simulink model "segway_PID2"  (R2020a)
settings: Solver=VariableStepAuto  StartTime=0.0  StopTime=60  RelTol=1e-3
undefined symbols (not defined in the file or in its folder): den1, den2, num1, num2
libraries: simulink x5
settings Model: Creator=santi  LastModifiedBy=santi

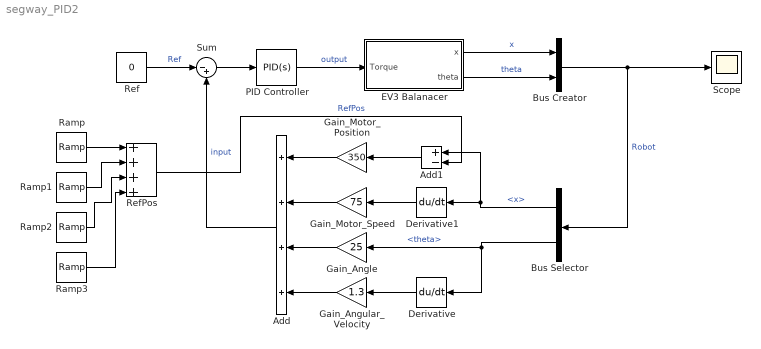
== system segway_PID2 ==
  Add : Sum  Inputs=++++
  Add1 : Sum  Inputs=+-
  Bus Creator : BusCreator  Inputs=2
  Bus Selector : BusSelector  OutputSignals=x,theta
  Derivative : Derivative
  Derivative1 : Derivative
  EV3 Balanacer : Subsystem
  Gain_Angle : Gain  Gain=25
  Gain_Angular_Velocity : Gain  Gain=1.3
  Gain_Motor_Position : Gain  Gain=350
  Gain_Motor_Speed : Gain  Gain=75
  PID Controller : simulink/Continuous/PID Controller  Controller=PID  Form=Parallel  TimeDomain=Continuous-time  UseExternalTs=off  SampleTime=-1  IntegratorMethod=Forward Euler  FilterMethod=Forward Euler  ControllerParametersSource=internal  P=0.6  I=14  D=0.005  UseFilter=on  N=100  TunerSelectOption=Transfer Function Based (PID Tuner App)  InitialConditionSource=internal  InitialConditionForIntegrator=0  InitialConditionForFilter=0  DifferentiatorICPrevScaledInput=0  ExternalReset=none  TrackingMode=off  Kt=1  LimitOutput=off  UpperSaturationLimit=inf  LowerSaturationLimit=-inf  LinearizeAsGain=on  AntiWindupMode=none  Kb=1  POutMin=[]  POutMax=[]  IOutMin=[]  IOutMax=[]  DOutMin=[]  DOutMax=[]  NOutMin=[]  NOutMax=[]  SumOutMin=[]  SumOutMax=[]  SaturationOutMin=[]  SaturationOutMax=[]  PParamMin=[]  PParamMax=[]  IParamMin=[]  IParamMax=[]  DParamMin=[]  DParamMax=[]  NParamMin=[]  NParamMax=[]  KbParamMin=[]  KbParamMax=[]  KtParamMin=[]  KtParamMax=[]  KbOutMin=[]  KbOutMax=[]  KtOutMin=[]  KtOutMax=[]  IntegratorOutMin=[]  IntegratorOutMax=[]  FilterOutMin=[]  FilterOutMax=[]  SumI1OutMin=[]  SumI1OutMax=[]  SumI2OutMin=[]  SumI2OutMax=[]  SumI3OutMin=[]  SumI3OutMax=[]  SumI4OutMin=[]  SumI4OutMax=[]  SumDOutMin=[]  SumDOutMax=[]  DifferentiatorOutMin=[]  DifferentiatorOutMax=[]  FilterDiffOutCoefMin=[]  FilterDiffOutCoefMax=[]  ReciprocalOutMin=[]  ReciprocalOutMax=[]  SumDenOutMin=[]  SumDenOutMax=[]  SumNumOutMin=[]  SumNumOutMax=[]  DivideOutMin=[]  DivideOutMax=[]  UdiffTsProdOutMin=[]  UdiffTsProdOutMax=[]  NTsProdOutMin=[]  NTsProdOutMax=[]  UintegralTsProdOutMin=[]  UintegralTsProdOutMax=[]  UngainTsProdOutMin=[]  UngainTsProdOutMax=[]  IntegratorContinuousStateAttributes=''  IntegratorStateMustResolveToSignalObject=off  IntegratorRTWStateStorageClass=Auto  FilterContinuousStateAttributes=''  FilterStateMustResolveToSignalObject=off  FilterRTWStateStorageClass=Auto  ParallelPVariant=InternalParameters  IdealPVariant=Disabled  IVariant=InternalParameters  DVariant=InternalParameters  IntegratorVariant=Continuous  SatVariant=Disabled  AWVariant=Passthrough  PCopyVariant=Disabled  TRVariant=Disabled  FdbkBlocksVariant=Forward  IdealPFdbkVariant=Disabled  SatFdbkVariant=Disabled  DerivativeFilterVariant=ContFilter  NVariant=InternalParameters  NCopyVariant=Disabled  FilterICVariant=InternalICsFilter  IntegratorICVariant=InternalICs  ExternalResetVariant=Disabled  TRSumVariant=Passthrough  SumFdbkVariant=Disabled  SumVariant=Sum_PID  TsampFilterVariant=InternalTs  TsampNgainVariant=Passthrough  TsampIntegralVariant=Passthrough
  Ramp : simulink/Sources/Ramp  slope=0.1  start=1  InitialOutput=0
  Ramp1 : simulink/Sources/Ramp  slope=-0.1  start=11  InitialOutput=0
  Ramp2 : simulink/Sources/Ramp  slope=-0.1  start=26  InitialOutput=0
  Ramp3 : simulink/Sources/Ramp  slope=0.1  start=36  InitialOutput=0
  Ref : Constant  Value=0
  RefPos : Sum  Inputs=++++
  Scope : Scope
  Sum : Sum  Inputs=|-+
  wires:
  EV3 Balanacer/1(x) -> Bus Creator/1  "x"
  EV3 Balanacer/2(theta) -> Bus Creator/2  "theta"
  Bus Creator/1 -> Bus Selector/1, Scope/1  "Robot"
  Sum/1 -> PID Controller/1
  Add/1 -> Sum/2  "input"
  Ref/1 -> Sum/1  "Ref"
  PID Controller/1 -> EV3 Balanacer/1(Torque)  "output"
  Gain_Motor_Position/1 -> Add/1
  Gain_Motor_Speed/1 -> Add/2
  Gain_Angle/1 -> Add/3
  Gain_Angular_Velocity/1 -> Add/4
  Derivative/1 -> Gain_Angular_Velocity/1
  Derivative1/1 -> Gain_Motor_Speed/1
  Bus Selector/1 -> Add1/1, Derivative1/1  "<x>"
  Bus Selector/2 -> Derivative/1, Gain_Angle/1  "<theta>"
  Add1/1 -> Gain_Motor_Position/1
  Ramp/1 -> RefPos/1
  Ramp1/1 -> RefPos/2
  Ramp2/1 -> RefPos/3
  Ramp3/1 -> RefPos/4
  RefPos/1 -> Add1/2  "RefPos"

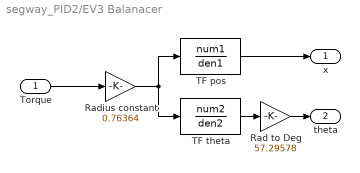
== system segway_PID2/EV3 Balanacer ==
  Torque : Inport
  Rad to Deg : Gain  Gain=57.29578
  Radius constant : Gain  Gain=0.76364
  TF pos : TransferFcn  Numerator=num1  Denominator=den1
  TF theta : TransferFcn  Numerator=num2  Denominator=den2
  x : Outport
  theta : Outport  Port=2
  wires:
  TF pos/1 -> x/1
  TF theta/1 -> Rad to Deg/1
  Rad to Deg/1 -> theta/1
  Torque/1 -> Radius constant/1
  Radius constant/1 -> TF pos/1, TF theta/1
